simulink model "EKF"  (Simulink 8.0)
settings: Solver=ode1  StartTime=0.0  StopTime=Inf  FixedStep=0.001  RelTol=1e-3
undefined symbols (not defined in the file or in its folder): d_p1, d_p2, g, l_1, l_2, m_1, m_2, m_3, P, Q, R, T, x0
settings Model: Creator=Bosselmann  LastModifiedBy=Bosselmann  BufferReuse=off
settings OptimizationCC: BlockReduction=off  OptimizeBlockIOStorage=off  BufferReuse=off  ExpressionFolding=off  LocalBlockOutputs=off
settings HardwareCC: ProdIntDivRoundTo=Zero  ProdEndianess=BigEndian  ProdHWDeviceType=Generic->Custom  TargetIntDivRoundTo=Zero  TargetEndianess=BigEndian  TargetHWDeviceType=Generic->Custom
settings RTWCC: SystemTargetFile=rti1401.tlc  MakeCommand=make_rti  TemplateMakefile=rti1401.tmf  Description=dSPACE DS1401 Hardware Platform  ProcessScript=rti1401_make_rtw_hook
settings STFCustomTargetCC: CodeReplacementLibrary=ANSI_C  ParMdlRefBuildCompliant=on  GeneratePreprocessorConditionals=Disable all  MatFileLogging=on  SystemTargetFile=rti1401.tlc
settings GRTTargetCC: CompOptLevelCompliant=off  ConcurrentExecutionCompliant=off  CombineOutputUpdateFcns=off  GRTInterface=on
settings CustomProperty: DataType=RTWOptions_EnumType_C__Program Files (x86)_dSPACE RCPHIL 74_MATLAB_RTI_RTI1401_TLC_rti1401_1InitialSimState  Value=RUN
settings EnumStrPairs: String=RUN

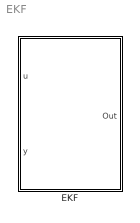
== system EKF ==
  EKF : Subsystem

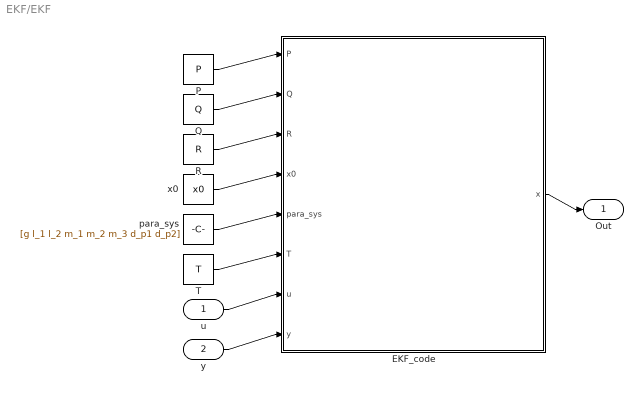
== system EKF/EKF ==
  u : Inport
  y : Inport  Port=2
  EKF_code : MATLAB Function  TreatAsAtomicUnit=on
  P : Constant  Value=P
  Q : Constant  Value=Q
  R : Constant  Value=R
  T : Constant  Value=T
  para_sys : Constant  Value=[g l_1 l_2 m_1 m_2 m_3 d_p1 d_p2]
  x0 : Constant  Value=x0
  Out : Outport
  wires:
  P/1 -> EKF_code/1(P)
  Q/1 -> EKF_code/2(Q)
  R/1 -> EKF_code/3(R)
  x0/1 -> EKF_code/4(x0)
  para_sys/1 -> EKF_code/5(para_sys)
  T/1 -> EKF_code/6(T)
  u/1 -> EKF_code/7(u)
  y/1 -> EKF_code/8(y)
  EKF_code/1(x) -> Out/1

== matlab function EKF/EKF_code ==
  data: P input double; Q input double; R input double; x0 input double; para_sys input double; T input double; u input double; y input double; x output double
function x  = extended_kalman_filter(P, Q, R, x0, para_sys, T, u, y)
% Extended Kalman Filter (EKF) fuer nichtlineare Systeme
% Das Extended Kalman Filter praediziert den Zustand eines nichtlinearen
% Systems durch Linearisierung im Arbeistpunkt.
% R ist die Kovarianzmatrix fuer das Messrauschen.
% Q ist die Kovarianzmatrix fuer das Prozessrauschen.
% Das Verhaeltnis von Q und R gibt die Dynamik des Filters vor.

persistent x_p P_p
% Parameter

g = para_sys(1);
l_1 = para_sys(2);
l_2 = para_sys(3);
m_1 = para_sys(4);
m_2 = para_sys(5);
m_3 = para_sys(6);
d_p1 = para_sys(7);
d_p2 = para_sys(8);

if isempty(x_p)
   x_p = x0;
   P_p = P;
   x = x_p;
else
%% Discrete Kalman filter time update equations

 x_1 = x_p(1);
 x_2 = x_p(2);
 x_3 = x_p(3);
 x_4 = x_p(4);

x = [x_1 + T*x_2;x_2 + (T*(12*d_p2*l_2*x_4 - 12*d_p1*l_2*x_2 - 12*d_p2*l_2*x_2 - cos(x_1 - x_3)*(18*d_p2*l_1*x_2 - 18*d_p2*l_1*x_4 + 9*l_1*l_2*m_2*u*cos(x_3) + 9*g*l_1*l_2*m_2*sin(x_3) + 9*l_1^2*l_2*m_2*x_2^2*sin(x_1 - x_3)) + 6*l_1*l_2*m_1*u*cos(x_1) + 12*l_1*l_2*m_2*u*cos(x_1) + 12*l_1*l_2*m_3*u*cos(x_1) + 6*g*l_1*l_2*m_1*sin(x_1) + 12*g*l_1*l_2*m_2*sin(x_1) + 12*g*l_1*l_2*m_3*sin(x_1) - 6*l_1*l_2^2*m_2*x_4^2*sin(x_1 - x_3)))/(l_1^2*l_2*(4*m_1 + 12*m_2 + 12*m_3 - 9*m_2*cos(x_1 - x_3)^2));x_3 + T*x_4;x_4 + (T*(sin(x_1 - x_3)*(36*l_1^2*l_2*m_2^2*x_2^2 + 12*l_1^2*l_2*m_1*m_2*x_2^2 + 36*l_1^2*l_2*m_2*m_3*x_2^2) + 24*d_p2*l_1*m_1*x_2 + 72*d_p2*l_1*m_2*x_2 - 24*d_p2*l_1*m_1*x_4 + 72*d_p2*l_1*m_3*x_2 - 72*d_p2*l_1*m_2*x_4 - 72*d_p2*l_1*m_3*x_4 + 36*d_p1*l_2*m_2*x_2*cos(x_1 - x_3) + 36*d_p2*l_2*m_2*x_2*cos(x_1 - x_3) - 36*d_p2*l_2*m_2*x_4*cos(x_1 - x_3) + 18*l_1*l_2*m_2^2*u*cos(x_3) + 18*g*l_1*l_2*m_2^2*sin(x_3) + 9*l_1*l_2^2*m_2^2*x_4^2*sin(2*x_1 - 2*x_3) - 18*l_1*l_2*m_2^2*u*cos(2*x_1 - x_3) - 18*g*l_1*l_2*m_2^2*sin(2*x_1 - x_3) + 3*l_1*l_2*m_1*m_2*u*cos(x_3) + 18*l_1*l_2*m_2*m_3*u*cos(x_3) + 3*g*l_1*l_2*m_1*m_2*sin(x_3) + 18*g*l_1*l_2*m_2*m_3*sin(x_3) - 9*l_1*l_2*m_1*m_2*u*cos(2*x_1 - x_3) - 18*l_1*l_2*m_2*m_3*u*cos(2*x_1 - x_3) - 9*g*l_1*l_2*m_1*m_2*sin(2*x_1 - x_3) - 18*g*l_1*l_2*m_2*m_3*sin(2*x_1 - x_3)))/(l_1*l_2^2*m_2*(8*m_1 + 15*m_2 + 24*m_3 - 9*m_2*cos(2*x_1 - 2*x_3)))];
       
        % Jacobian Matrix
A = [1, T, 0, 0;- (T*(6*l_1*l_2*m_1*u*sin(x_1) - sin(x_1 - x_3)*(18*d_p2*l_1*x_2 - 18*d_p2*l_1*x_4 + 9*l_1*l_2*m_2*u*cos(x_3) + 9*g*l_1*l_2*m_2*sin(x_3) + 9*l_1^2*l_2*m_2*x_2^2*sin(x_1 - x_3)) + 12*l_1*l_2*m_2*u*sin(x_1) + 12*l_1*l_2*m_3*u*sin(x_1) + 9*l_1^2*l_2*m_2*x_2^2*cos(x_1 - x_3)^2 - 6*g*l_1*l_2*m_1*cos(x_1) - 12*g*l_1*l_2*m_2*cos(x_1) - 12*g*l_1*l_2*m_3*cos(x_1) + 6*l_1*l_2^2*m_2*x_4^2*cos(x_1 - x_3)))/(l_1^2*l_2*(4*m_1 + 12*m_2 + 12*m_3 - 9*m_2*cos(x_1 - x_3)^2)) - (18*T*m_2*cos(x_1 - x_3)*sin(x_1 - x_3)*(12*d_p2*l_2*x_4 - 12*d_p1*l_2*x_2 - 12*d_p2*l_2*x_2 - cos(x_1 - x_3)*(18*d_p2*l_1*x_2 - 18*d_p2*l_1*x_4 + 9*l_1*l_2*m_2*u*cos(x_3) + 9*g*l_1*l_2*m_2*sin(x_3) + 9*l_1^2*l_2*m_2*x_2^2*sin(x_1 - x_3)) + 6*l_1*l_2*m_1*u*cos(x_1) + 12*l_1*l_2*m_2*u*cos(x_1) + 12*l_1*l_2*m_3*u*cos(x_1) + 6*g*l_1*l_2*m_1*sin(x_1) + 12*g*l_1*l_2*m_2*sin(x_1) + 12*g*l_1*l_2*m_3*sin(x_1) - 6*l_1*l_2^2*m_2*x_4^2*sin(x_1 - x_3)))/(l_1^2*l_2*(4*m_1 + 12*m_2 + 12*m_3 - 9*m_2*cos(x_1 - x_3)^2)^2), 1 - (T*(12*d_p1*l_2 + 12*d_p2*l_2 + cos(x_1 - x_3)*(18*d_p2*l_1 + 18*l_1^2*l_2*m_2*x_2*sin(x_1 - x_3))))/(l_1^2*l_2*(4*m_1 + 12*m_2 + 12*m_3 - 9*m_2*cos(x_1 - x_3)^2)), (T*(cos(x_1 - x_3)*(9*l_1*l_2*m_2*u*sin(x_3) - 9*g*l_1*l_2*m_2*cos(x_3) + 9*l_1^2*l_2*m_2*x_2^2*cos(x_1 - x_3)) - sin(x_1 - x_3)*(18*d_p2*l_1*x_2 - 18*d_p2*l_1*x_4 + 9*l_1*l_2*m_2*u*cos(x_3) + 9*g*l_1*l_2*m_2*sin(x_3) + 9*l_1^2*l_2*m_2*x_2^2*sin(x_1 - x_3)) + 6*l_1*l_2^2*m_2*x_4^2*cos(x_1 - x_3)))/(l_1^2*l_2*(4*m_1 + 12*m_2 + 12*m_3 - 9*m_2*cos(x_1 - x_3)^2)) + (18*T*m_2*cos(x_1 - x_3)*sin(x_1 - x_3)*(12*d_p2*l_2*x_4 - 12*d_p1*l_2*x_2 - 12*d_p2*l_2*x_2 - cos(x_1 - x_3)*(18*d_p2*l_1*x_2 - 18*d_p2*l_1*x_4 + 9*l_1*l_2*m_2*u*cos(x_3) + 9*g*l_1*l_2*m_2*sin(x_3) + 9*l_1^2*l_2*m_2*x_2^2*sin(x_1 - x_3)) + 6*l_1*l_2*m_1*u*cos(x_1) + 12*l_1*l_2*m_2*u*cos(x_1) + 12*l_1*l_2*m_3*u*cos(x_1) + 6*g*l_1*l_2*m_1*sin(x_1) + 12*g*l_1*l_2*m_2*sin(x_1) + 12*g*l_1*l_2*m_3*sin(x_1) - 6*l_1*l_2^2*m_2*x_4^2*sin(x_1 - x_3)))/(l_1^2*l_2*(4*m_1 + 12*m_2 + 12*m_3 - 9*m_2*cos(x_1 - x_3)^2)^2), (T*(12*d_p2*l_2 + 18*d_p2*l_1*cos(x_1 - x_3) - 12*l_1*l_2^2*m_2*x_4*sin(x_1 - x_3)))/(l_1^2*l_2*(4*m_1 + 12*m_2 + 12*m_3 - 9*m_2*cos(x_1 - x_3)^2));0, 0, 1, T;(T*(cos(x_1 - x_3)*(36*l_1^2*l_2*m_2^2*x_2^2 + 12*l_1^2*l_2*m_1*m_2*x_2^2 + 36*l_1^2*l_2*m_2*m_3*x_2^2) - 36*d_p1*l_2*m_2*x_2*sin(x_1 - x_3) - 36*d_p2*l_2*m_2*x_2*sin(x_1 - x_3) + 36*d_p2*l_2*m_2*x_4*sin(x_1 - x_3) + 18*l_1*l_2^2*m_2^2*x_4^2*cos(2*x_1 - 2*x_3) - 36*g*l_1*l_2*m_2^2*cos(2*x_1 - x_3) + 36*l_1*l_2*m_2^2*u*sin(2*x_1 - x_3) + 18*l_1*l_2*m_1*m_2*u*sin(2*x_1 - x_3) + 36*l_1*l_2*m_2*m_3*u*sin(2*x_1 - x_3) - 18*g*l_1*l_2*m_1*m_2*cos(2*x_1 - x_3) - 36*g*l_1*l_2*m_2*m_3*cos(2*x_1 - x_3)))/(l_1*l_2^2*m_2*(8*m_1 + 15*m_2 + 24*m_3 - 9*m_2*cos(2*x_1 - 2*x_3))) - (18*T*sin(2*x_1 - 2*x_3)*(sin(x_1 - x_3)*(36*l_1^2*l_2*m_2^2*x_2^2 + 12*l_1^2*l_2*m_1*m_2*x_2^2 + 36*l_1^2*l_2*m_2*m_3*x_2^2) + 24*d_p2*l_1*m_1*x_2 + 72*d_p2*l_1*m_2*x_2 - 24*d_p2*l_1*m_1*x_4 + 72*d_p2*l_1*m_3*x_2 - 72*d_p2*l_1*m_2*x_4 - 72*d_p2*l_1*m_3*x_4 + 36*d_p1*l_2*m_2*x_2*cos(x_1 - x_3) + 36*d_p2*l_2*m_2*x_2*cos(x_1 - x_3) - 36*d_p2*l_2*m_2*x_4*cos(x_1 - x_3) + 18*l_1*l_2*m_2^2*u*cos(x_3) + 18*g*l_1*l_2*m_2^2*sin(x_3) + 9*l_1*l_2^2*m_2^2*x_4^2*sin(2*x_1 - 2*x_3) - 18*l_1*l_2*m_2^2*u*cos(2*x_1 - x_3) - 18*g*l_1*l_2*m_2^2*sin(2*x_1 - x_3) + 3*l_1*l_2*m_1*m_2*u*cos(x_3) + 18*l_1*l_2*m_2*m_3*u*cos(x_3) + 3*g*l_1*l_2*m_1*m_2*sin(x_3) + 18*g*l_1*l_2*m_2*m_3*sin(x_3) - 9*l_1*l_2*m_1*m_2*u*cos(2*x_1 - x_3) - 18*l_1*l_2*m_2*m_3*u*cos(2*x_1 - x_3) - 9*g*l_1*l_2*m_1*m_2*sin(2*x_1 - x_3) - 18*g*l_1*l_2*m_2*m_3*sin(2*x_1 - x_3)))/(l_1*l_2^2*(8*m_1 + 15*m_2 + 24*m_3 - 9*m_2*cos(2*x_1 - 2*x_3))^2), (T*(sin(x_1 - x_3)*(72*l_1^2*l_2*m_2^2*x_2 + 24*l_1^2*l_2*m_1*m_2*x_2 + 72*l_1^2*l_2*m_2*m_3*x_2) + 24*d_p2*l_1*m_1 + 72*d_p2*l_1*m_2 + 72*d_p2*l_1*m_3 + 36*d_p1*l_2*m_2*cos(x_1 - x_3) + 36*d_p2*l_2*m_2*cos(x_1 - x_3)))/(l_1*l_2^2*m_2*(8*m_1 + 15*m_2 + 24*m_3 - 9*m_2*cos(2*x_1 - 2*x_3))), (18*T*sin(2*x_1 - 2*x_3)*(sin(x_1 - x_3)*(36*l_1^2*l_2*m_2^2*x_2^2 + 12*l_1^2*l_2*m_1*m_2*x_2^2 + 36*l_1^2*l_2*m_2*m_3*x_2^2) + 24*d_p2*l_1*m_1*x_2 + 72*d_p2*l_1*m_2*x_2 - 24*d_p2*l_1*m_1*x_4 + 72*d_p2*l_1*m_3*x_2 - 72*d_p2*l_1*m_2*x_4 - 72*d_p2*l_1*m_3*x_4 + 36*d_p1*l_2*m_2*x_2*cos(x_1 - x_3) + 36*d_p2*l_2*m_2*x_2*cos(x_1 - x_3) - 36*d_p2*l_2*m_2*x_4*cos(x_1 - x_3) + 18*l_1*l_2*m_2^2*u*cos(x_3) + 18*g*l_1*l_2*m_2^2*sin(x_3) + 9*l_1*l_2^2*m_2^2*x_4^2*sin(2*x_1 - 2*x_3) - 18*l_1*l_2*m_2^2*u*cos(2*x_1 - x_3) - 18*g*l_1*l_2*m_2^2*sin(2*x_1 - x_3) + 3*l_1*l_2*m_1*m_2*u*cos(x_3) + 18*l_1*l_2*m_2*m_3*u*cos(x_3) + 3*g*l_1*l_2*m_1*m_2*sin(x_3) + 18*g*l_1*l_2*m_2*m_3*sin(x_3) - 9*l_1*l_2*m_1*m_2*u*cos(2*x_1 - x_3) - 18*l_1*l_2*m_2*m_3*u*cos(2*x_1 - x_3) - 9*g*l_1*l_2*m_1*m_2*sin(2*x_1 - x_3) - 18*g*l_1*l_2*m_2*m_3*sin(2*x_1 - x_3)))/(l_1*l_2^2*(8*m_1 + 15*m_2 + 24*m_3 - 9*m_2*cos(2*x_1 - 2*x_3))^2) - (T*(cos(x_1 - x_3)*(36*l_1^2*l_2*m_2^2*x_2^2 + 12*l_1^2*l_2*m_1*m_2*x_2^2 + 36*l_1^2*l_2*m_2*m_3*x_2^2) - 36*d_p1*l_2*m_2*x_2*sin(x_1 - x_3) - 36*d_p2*l_2*m_2*x_2*sin(x_1 - x_3) + 36*d_p2*l_2*m_2*x_4*sin(x_1 - x_3) - 18*g*l_1*l_2*m_2^2*cos(x_3) + 18*l_1*l_2*m_2^2*u*sin(x_3) + 18*l_1*l_2^2*m_2^2*x_4^2*cos(2*x_1 - 2*x_3) - 18*g*l_1*l_2*m_2^2*cos(2*x_1 - x_3) + 18*l_1*l_2*m_2^2*u*sin(2*x_1 - x_3) + 9*l_1*l_2*m_1*m_2*u*sin(2*x_1 - x_3) + 18*l_1*l_2*m_2*m_3*u*sin(2*x_1 - x_3) - 3*g*l_1*l_2*m_1*m_2*cos(x_3) - 18*g*l_1*l_2*m_2*m_3*cos(x_3) + 3*l_1*l_2*m_1*m_2*u*sin(x_3) + 18*l_1*l_2*m_2*m_3*u*sin(x_3) - 9*g*l_1*l_2*m_1*m_2*cos(2*x_1 - x_3) - 18*g*l_1*l_2*m_2*m_3*cos(2*x_1 - x_3)))/(l_1*l_2^2*m_2*(8*m_1 + 15*m_2 + 24*m_3 - 9*m_2*cos(2*x_1 - 2*x_3))), 1 - (T*(24*d_p2*l_1*m_1 + 72*d_p2*l_1*m_2 + 72*d_p2*l_1*m_3 + 36*d_p2*l_2*m_2*cos(x_1 - x_3) - 18*l_1*l_2^2*m_2^2*x_4*sin(2*x_1 - 2*x_3)))/(l_1*l_2^2*m_2*(8*m_1 + 15*m_2 + 24*m_3 - 9*m_2*cos(2*x_1 - 2*x_3)))];
C = [1 0 0 0];

%% Discrete Kalman filter measurement update equations
P   = A * P_p * A' + Q;
K   = P * C'/( C * P * C' + R);
x   = x + (K * (y - C * x));
P_p  = (eye(size(A)) - K * C) * P;
x_p  = x;
end
